simulink model "bldc_model_bst"  (R2014b)
settings: Solver=ode4  StartTime=0.0  StopTime=72  FixedStep=0.01  RelTol=1e-3
values from neighbouring files (symbols this model uses):
  km = 1/ki    (= 0.01039998336)    [rwa05.m]
undefined symbols (not defined in the file or in its folder): spd_0
libraries: simulink x2
settings Model: Creator=root  LastModifiedBy=root

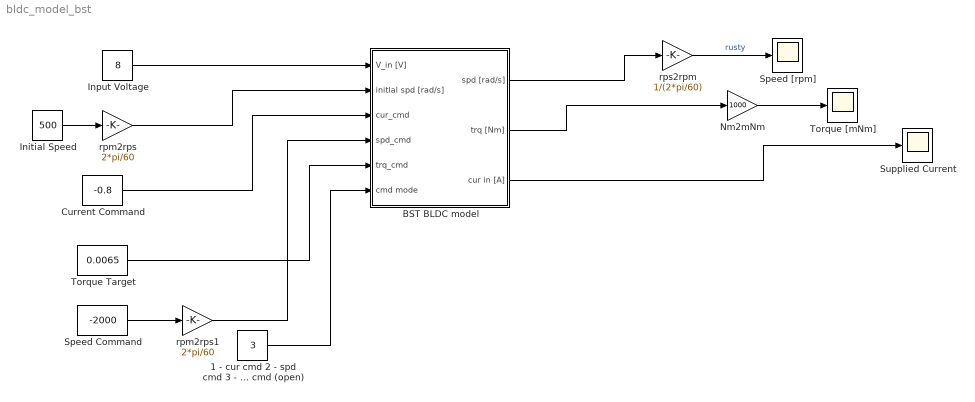
== system bldc_model_bst ==
  1 - cur cmd 2 - spd cmd 3 - trq cmd 4 - trq cmd (open) : Constant  Value=3
  BST BLDC model : Subsystem  mask{Ke=1.026E-3/(2*pi/60), Km=1/96.154, R=2.3, frctn_c=[-3.77e-09, -1.42e-06, -6.76e-04], frctn_p=[-3.39e-09, -1.57e-06, -5.89e-04], frctn_n=[-9.44e-09, -4.31e-05, +3.57e-04], J=978.548e-6, i_max=0.9, V_in=8.0}
      mask prompts: Ke "Back-EMF Constant [V/(rad/s)]"; Km "Motor Torque Constant [Nm/A]"; R "Motor Resistance [Ohm]"; frctn_c "Friction Coefficients"; frctn_p "Friction Coefficients Pos"; frctn_n "Friction Coefficients Neg"; J "Moment of Inertia [kgm2]"; i_max "Maximum Current [A]"; V_in "Input Voltage [V]"
  "Current Command " : Constant  Value=-0.8
  Initial Speed : Constant  Value=500
  Input Voltage : Constant  Value=8
  Nm2mNm : Gain  Gain=1000
  Speed Command : Constant  Value=-2000
  "Speed [rpm] " : Scope
      settings: ShowLegends=on  TimeRange=30  YMin=-3000  YMax=2000
  Supplied Current : Scope
      settings: ShowLegends=on  TimeRange=10  YMin=0.344  YMax=0.351  SaveName=ScopeData2
  Torque Target : Constant  Value=0.0065
  Torque [mNm] : Scope
      settings: ShowLegends=on  TimeRange=300  YMin=-20  YMax=20
  rpm2rps : Gain  Gain=2*pi/60
  rpm2rps1 : Gain  Gain=2*pi/60
  rps2rpm : Gain  Gain=1/(2*pi/60)
  wires:
  BST BLDC model/1(spd [rad/s]) -> rps2rpm/1
  rps2rpm/1 -> "Speed [rpm] "/1  "rusty"
  Input Voltage/1 -> BST BLDC model/1(V_in [V])
  Initial Speed/1 -> rpm2rps/1
  rpm2rps/1 -> BST BLDC model/2(initlal spd [rad/s])
  BST BLDC model/2(trq [Nm]) -> Nm2mNm/1
  Nm2mNm/1 -> Torque [mNm]/1
  BST BLDC model/3(cur in [A]) -> Supplied Current/1
  Speed Command/1 -> rpm2rps1/1
  "Current Command "/1 -> BST BLDC model/3(cur_cmd)
  1 - cur cmd 2 - spd cmd 3 - trq cmd 4 - trq cmd (open)/1 -> BST BLDC model/6(cmd mode)
  rpm2rps1/1 -> BST BLDC model/4(spd_cmd)
  Torque Target/1 -> BST BLDC model/5(trq_cmd)

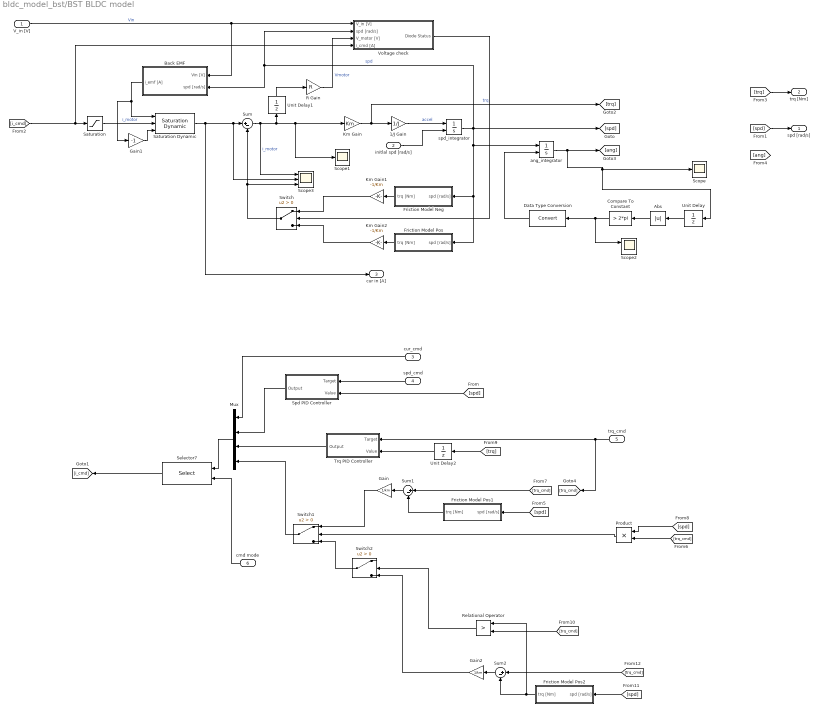
== system bldc_model_bst/BST BLDC model ==
  V_in [V] : Inport
  initlal spd [rad/s] : Inport  Port=2
  cur_cmd : Inport  Port=3
  spd_cmd : Inport  Port=4
  trq_cmd : Inport  Port=5
  cmd mode : Inport  Port=6
  1/J Gain : Gain  Gain=1/J
  Abs : Abs
  Back EMF : Subsystem
  Compare To Constant : simulink/Logic and Bit Operations/Compare To Constant  relop=>  const=2*pi  OutDataTypeStr=uint8
  Data Type Conversion : DataTypeConversion
  Friction Model Neg : Subsystem  mask{frctn=frctn_n}
      mask prompts: frctn "Friction Coefficients"
  Friction Model Pos : Subsystem  mask{frctn=frctn_p}
      mask prompts: frctn "Friction Coefficients"
  Friction Model Pos1 : Subsystem  mask{frctn=frctn_p}
      mask prompts: frctn "Friction Coefficients"
  Friction Model Pos2 : Subsystem  mask{frctn=frctn_p}
      mask prompts: frctn "Friction Coefficients"
  Gain : Gain  Gain=1/km
  Gain1 : Gain  Gain=-1
  Gain2 : Gain  Gain=1/km
  Km Gain : Gain  Gain=Km
  Km Gain1 : Gain  Gain=-1/Km
  Km Gain2 : Gain  Gain=-1/Km
  Mux : Mux
  Product : Product
  R Gain : Gain  Gain=R
  Relational Operator : RelationalOperator  Operator=>  OutDataTypeStr=boolean
  Saturation : Saturate  UpperLimit=i_max  LowerLimit=-i_max
  Saturation Dynamic : simulink/Discontinuities/Saturation Dynamic  OutMin=[]  OutMax=[]  OutDataTypeStr=Inherit: Same as second input  OutDataType=fixdt(1, 16)  OutScaling=2^-10  DoSatur=off
  Scope : Scope
      settings: TimeRange=30  SaveName=ScopeData3
  Scope1 : Scope
      settings: TimeRange=30  SaveName=ScopeData5
  Scope2 : Scope  NumInputPorts=2
      settings: TimeRange=30  YMin=-5~-5  YMax=5~5  SaveName=ScopeData7
  Scope3 : Scope  NumInputPorts=3
      settings: TimeRange=30  YMin=-5~-5~-5  YMax=5~5~5  SaveName=ScopeData8
  Selector7 : Selector  NumberOfDimensions=2  InputPortWidth=3  IndexOptions=Select all,Index vector (port)  Indices=[1 3],1  OutputSizes=1,1
  Spd PID Controller : Subsystem  mask{kp=100E-3, ki=3.0e-05, kd=0.0, aw_thr=0.9, aw_fact=0}
      mask prompts: kp "Proportional Gain"; ki "Integrator Gain"; kd "Derivative Gain"; aw_thr "AntiWindup Threshold"; aw_fact "AntiWindup Factor"
      mask DialogControl DescTextVar Prompt: This is a general PID controller with propotional gains, derivative gain and integral gain
  Sum : Sum  Inputs=|+-
  Sum1 : Sum  Inputs=|+-
  Sum2 : Sum  Inputs=|+-
  Switch : Switch  Criteria=u2 > Threshold
  Switch1 : Switch  Criteria=u2 > Threshold
  Switch2 : Switch  Criteria=u2 > Threshold
  Trq PID Controller : Subsystem  mask{kp=5.0, ki=0.03, kd=0.0, aw_thr=0.9, aw_fact=0}
      mask prompts: kp "Proportional Gain"; ki "Integrator Gain"; kd "Derivative Gain"; aw_thr "AntiWindup Threshold"; aw_fact "AntiWindup Factor"
      mask DialogControl DescTextVar Prompt: This is a general PID controller with propotional gains, derivative gain and integral gain
  Unit Delay : UnitDelay  SampleTime=-1
  Unit Delay1 : UnitDelay  SampleTime=-1
  Unit Delay2 : UnitDelay  SampleTime=-1
  Voltage check : Subsystem
  ang_integrator : Integrator  ExternalReset=rising
  spd_integrator : Integrator  InitialConditionSource=external  InitialCondition=spd_0
  spd [rad/s] : Outport
  trq [Nm] : Outport  Port=2
  cur in [A] : Outport  Port=3
  wires:
  Km Gain/1 -> [trq], 1/J Gain/1  "trq"
  spd_integrator/1 -> Voltage check/2(spd [rad/s]), Back EMF/2(spd [rad/s]), [spd], Friction Model Pos/1(spd [rad/s]), Friction Model Neg/1(spd [rad/s]), ang_integrator/1  "spd"
  Sum/1 -> Scope3/1, Scope1/1, Km Gain/1, Unit Delay1/1  "i_motor"
  [i_cmd] -> Voltage check/4(i_cmd [A]), Saturation/1
  Friction Model Neg/1(trq [Nm]) -> Km Gain1/1
  1/J Gain/1 -> spd_integrator/1  "accel"
  V_in [V]/1 -> Voltage check/1(V_in [V]), Back EMF/1(Vin [V])  "Vin"
  Saturation/1 -> Saturation Dynamic/2  "i_motor"
  Saturation Dynamic/1 -> cur in [A]/1, Scope3/2, Sum/1
  Gain1/1 -> Saturation Dynamic/3
  Friction Model Pos/1(trq [Nm]) -> Km Gain2/1
  Unit Delay1/1 -> R Gain/1
  Back EMF/1(i_emf [A]) -> Saturation Dynamic/1, Gain1/1
  Km Gain2/1 -> Switch/3
  Km Gain1/1 -> Switch/1
  Voltage check/1(Diode Status) -> Switch/2
  R Gain/1 -> Voltage check/3(V_motor [V])  "Vmotor"
  initlal spd [rad/s]/1 -> spd_integrator/2
  Abs/1 -> Compare To Constant/1
  ang_integrator/1 -> [ang], Scope/1, Unit Delay/1
  Unit Delay/1 -> Abs/1
  Data Type Conversion/1 -> ang_integrator/2
  Compare To Constant/1 -> Scope2/1, Data Type Conversion/1
  Switch/1 -> Scope3/3, Sum/2
  [spd] -> Spd PID Controller/2(Value)
  spd_cmd/1 -> Spd PID Controller/1(Target)
  [spd] -> spd [rad/s]/1
  [trq] -> trq [Nm]/1
  trq_cmd/1 -> Trq PID Controller/1(Target), [trq_cmd]
  Mux/1 -> Selector7/1
  Spd PID Controller/1(Output) -> Mux/2
  Selector7/1 -> [i_cmd]
  cmd mode/1 -> Selector7/2
  cur_cmd/1 -> Mux/1
  Sum1/1 -> Gain/1
  Friction Model Pos1/1(trq [Nm]) -> Sum1/2
  [spd] -> Friction Model Pos1/1(spd [rad/s])
  Gain/1 -> Switch1/1
  [trq_cmd] -> Sum1/1
  [trq_cmd] -> Product/2
  [spd] -> Product/1
  Product/1 -> Switch1/2
  Switch1/1 -> Mux/4
  Friction Model Pos2/1(trq [Nm]) -> Sum2/2, Relational Operator/1
  Switch2/1 -> Switch1/3
  [trq_cmd] -> Relational Operator/2
  Relational Operator/1 -> Switch2/2
  Sum2/1 -> Gain2/1
  [spd] -> Friction Model Pos2/1(spd [rad/s])
  Gain2/1 -> Switch2/3
  [trq_cmd] -> Sum2/1
  [trq] -> Unit Delay2/1
  Trq PID Controller/1(Output) -> Mux/3
  Unit Delay2/1 -> Trq PID Controller/2(Value)

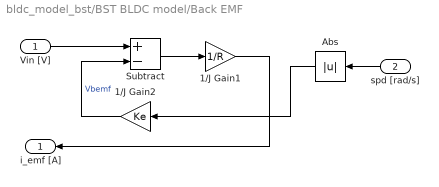
== system bldc_model_bst/BST BLDC model/Back EMF ==
  Vin [V] : Inport
  spd [rad/s] : Inport  Port=2
  1/J Gain1 : Gain  Gain=1/R
  1/J Gain2 : Gain  Gain=Ke
  Abs : Abs
  Subtract : Sum  Inputs=+-
  i_emf [A] : Outport
  wires:
  Vin [V]/1 -> Subtract/1
  1/J Gain1/1 -> i_emf [A]/1
  Subtract/1 -> 1/J Gain1/1
  spd [rad/s]/1 -> Abs/1
  1/J Gain2/1 -> Subtract/2  "Vbemf"
  Abs/1 -> 1/J Gain2/1

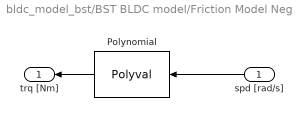
== system bldc_model_bst/BST BLDC model/Friction Model Neg ==
  spd [rad/s] : Inport
  Polynomial : Polyval  Coefs=frctn
  trq [Nm] : Outport
  wires:
  spd [rad/s]/1 -> Polynomial/1
  Polynomial/1 -> trq [Nm]/1

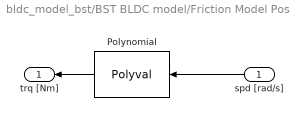
== system bldc_model_bst/BST BLDC model/Friction Model Pos ==
  spd [rad/s] : Inport
  Polynomial : Polyval  Coefs=frctn
  trq [Nm] : Outport
  wires:
  spd [rad/s]/1 -> Polynomial/1
  Polynomial/1 -> trq [Nm]/1

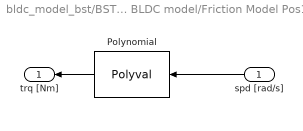
== system bldc_model_bst/BST BLDC model/Friction Model Pos1 ==
  spd [rad/s] : Inport
  Polynomial : Polyval  Coefs=frctn
  trq [Nm] : Outport
  wires:
  spd [rad/s]/1 -> Polynomial/1
  Polynomial/1 -> trq [Nm]/1

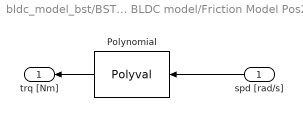
== system bldc_model_bst/BST BLDC model/Friction Model Pos2 ==
  spd [rad/s] : Inport
  Polynomial : Polyval  Coefs=frctn
  trq [Nm] : Outport
  wires:
  spd [rad/s]/1 -> Polynomial/1
  Polynomial/1 -> trq [Nm]/1

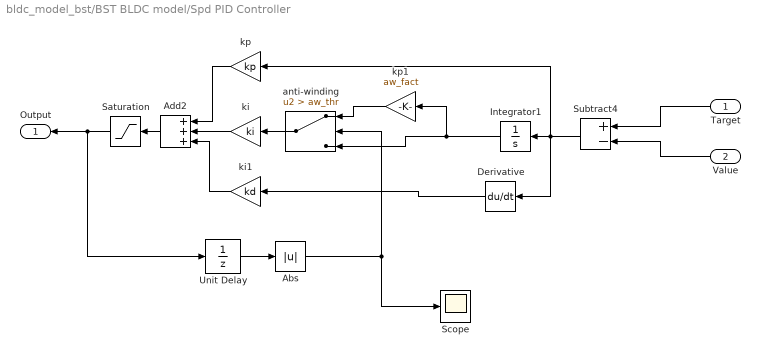
== system bldc_model_bst/BST BLDC model/Spd PID Controller ==
  Target : Inport
  Value : Inport  Port=2
  Abs : Abs
  Add2 : Sum  Inputs=+++
  Derivative : Derivative
  Integrator1 : Integrator
  Saturation : Saturate  UpperLimit=aw_thr  LowerLimit=-aw_thr
  Scope : Scope
      settings: SaveName=ScopeData6
  Subtract4 : Sum  Inputs=+-
  Unit Delay : UnitDelay  SampleTime=-1
  anti-winding : Switch  Criteria=u2 > Threshold  Threshold=aw_thr
  ki : Gain  Gain=ki
  ki1 : Gain  Gain=kd
  kp : Gain  Gain=kp
  kp1 : Gain  Gain=aw_fact
  Output : Outport
  wires:
  Target/1 -> Subtract4/1
  Value/1 -> Subtract4/2
  Integrator1/1 -> anti-winding/3, kp1/1
  kp/1 -> Add2/1
  ki/1 -> Add2/2
  Derivative/1 -> ki1/1
  ki1/1 -> Add2/3
  Subtract4/1 -> Integrator1/1, kp/1, Derivative/1
  anti-winding/1 -> ki/1
  kp1/1 -> anti-winding/1
  Abs/1 -> Scope/1, anti-winding/2
  Unit Delay/1 -> Abs/1
  Add2/1 -> Saturation/1
  Saturation/1 -> Output/1, Unit Delay/1

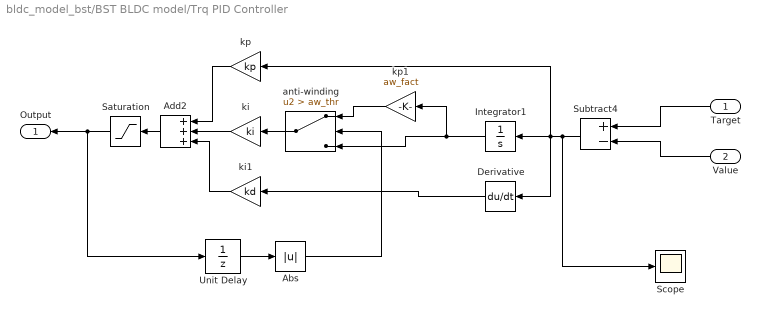
== system bldc_model_bst/BST BLDC model/Trq PID Controller ==
  Target : Inport
  Value : Inport  Port=2
  Abs : Abs
  Add2 : Sum  Inputs=+++
  Derivative : Derivative
  Integrator1 : Integrator
  Saturation : Saturate  UpperLimit=aw_thr  LowerLimit=-aw_thr
  Scope : Scope
      settings: SaveName=ScopeData6
  Subtract4 : Sum  Inputs=+-
  Unit Delay : UnitDelay  SampleTime=-1
  anti-winding : Switch  Criteria=u2 > Threshold  Threshold=aw_thr
  ki : Gain  Gain=ki
  ki1 : Gain  Gain=kd
  kp : Gain  Gain=kp
  kp1 : Gain  Gain=aw_fact
  Output : Outport
  wires:
  Target/1 -> Subtract4/1
  Value/1 -> Subtract4/2
  Integrator1/1 -> anti-winding/3, kp1/1
  kp/1 -> Add2/1
  ki/1 -> Add2/2
  Derivative/1 -> ki1/1
  ki1/1 -> Add2/3
  Subtract4/1 -> Scope/1, Integrator1/1, kp/1, Derivative/1
  anti-winding/1 -> ki/1
  kp1/1 -> anti-winding/1
  Abs/1 -> anti-winding/2
  Unit Delay/1 -> Abs/1
  Add2/1 -> Saturation/1
  Saturation/1 -> Output/1, Unit Delay/1

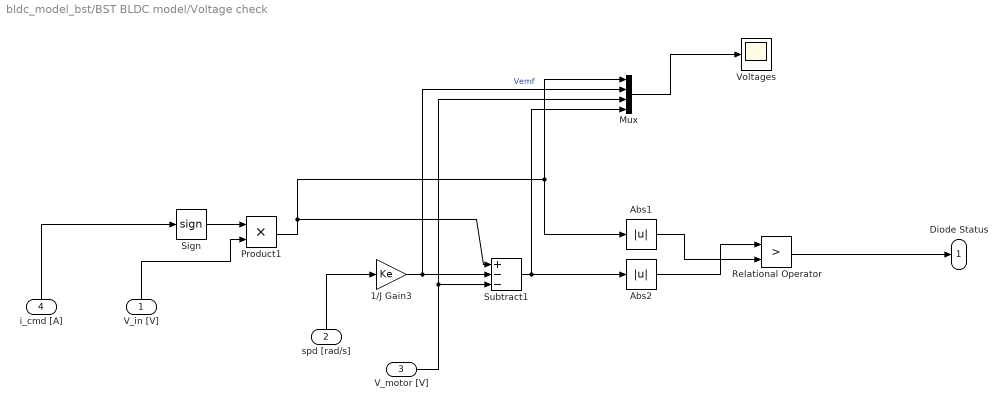
== system bldc_model_bst/BST BLDC model/Voltage check ==
  V_in [V] : Inport
  spd [rad/s] : Inport  Port=2
  V_motor [V] : Inport  Port=3
  i_cmd [A] : Inport  Port=4
  1/J Gain3 : Gain  Gain=Ke
  Abs1 : Abs
  Abs2 : Abs
  Mux : Mux
  Product1 : Product
  Relational Operator : RelationalOperator  Operator=>  OutDataTypeStr=boolean
  Sign : Signum
  Subtract1 : Sum  Inputs=+--
  Voltages : Scope
      settings: ShowLegends=on  TimeRange=30  YMin=-25  YMax=0  SaveName=ScopeData4  ScrollMode=on
  Diode Status : Outport
  wires:
  spd [rad/s]/1 -> 1/J Gain3/1
  Relational Operator/1 -> Diode Status/1
  1/J Gain3/1 -> Mux/2, Subtract1/2  "Vemf"
  Sign/1 -> Product1/1
  Subtract1/1 -> Mux/4, Abs2/1
  Abs2/1 -> Relational Operator/1
  V_motor [V]/1 -> Mux/3, Subtract1/3
  i_cmd [A]/1 -> Sign/1
  Abs1/1 -> Relational Operator/2
  V_in [V]/1 -> Product1/2
  Mux/1 -> Voltages/1
  Product1/1 -> Abs1/1, Mux/1, Subtract1/1
